simulink model "edma_scatter_gather_transfer_s32k14x"  (Simulink 9.0)
settings: Solver=FixedStepDiscrete  StartTime=0.0  StopTime=10.0  FixedStep=0.5  RelTol=1e-3  EnableMultiTasking=on
InitFcn:
  | mbd_s32k_consistency_checks(bdroot(gcs));
undefined symbols (not defined in the file): LQFP
libraries: mbd_s32k1xx_ec_toolbox x6, simulink x1
Description:
  | Press SW3 to trigger an eDMA transfer to PTOR register; this toggles PTD0 and PTD15,
  | thus blinking the red and blue LEDs.
  | 
  | Press SW2 to trigger eDMA transfer continuously (at every step). Pressing it again will stop this process.
  | 
  | Verification:
  | LED blink (purple) at every SW3 press.
  | LED blinks continuously at 0.5s after pressing SW2.
settings Model: Creator=NXP MBDT Team  LastModifiedBy=nxf35172
settings DataIOCC: ExternalInput=off  InitialState=off  LimitDataPoints=on  SaveFormat=Dataset  SaveOutput=off  SignalLogging=off  SaveTime=off
settings OptimizationCC: DefaultParameterBehavior=Inlined  PassReuseOutputArgsAs=Individual arguments  LifeSpan=auto
settings DebuggingCC: UnderspecifiedInitializationDetection=Simplified  MergeDetectMultiDrivingBlocksExec=error  InheritedTsInSrcMsg=none  SingleTaskRateTransMsg=error  ParameterTunabilityLossMsg=error  UnconnectedInputMsg=error  UnconnectedOutputMsg=error  UnconnectedLineMsg=error  AllowSymbolicDim=off  UnknownTsInhSupMsg=error
settings HardwareCC: ProdLargestAtomicInteger=Long  ProdLargestAtomicFloat=Double  ProdIntDivRoundTo=Zero  ProdEndianess=LittleEndian  ProdHWDeviceType=ARM Compatible->ARM Cortex
settings SFSimCC: MATLABDynamicMemAlloc=off
settings RTWCC: SystemTargetFile=mbd_s32k.tlc  MakeCommand=mbd_s32k_make_rtw COPY_MDLREF_INCLUDES=0  TemplateMakefile=mbd_s32k.tmf  Description=Model Based Design Toolbox S32K14x Code Generation Target  GenerateReport=on  IncludeHyperlinkInReport=on  LaunchReport=on  GenerateTraceInfo=on  GenerateTraceReport=on  GenerateTraceReportSl=on  GenerateTraceReportSf=on  GenerateTraceReportEml=on
settings CodeAppCC: ForceParamTrailComments=on  IgnoreCustomStorageClasses=off  OperatorAnnotations=on  SimulinkDataObjDesc=on  SFDataObjDesc=on  InsertBlockDesc=on  StateflowObjectComments=off
settings STFCustomTargetCC: MultiwordLength=256  ModelReferenceCompliant=off  CombineOutputUpdateFcns=on  ERTCustomFileBanners=on  SupportContinuousTime=off  SupportNonInlinedSFcns=off  RemoveResetFunc=on  MATLABClassNameForMDSCustomization=Simulink.SoftwareTarget.ERTCustomization  GRTInterface=off  SystemTargetFile=mbd_s32k.tlc
settings ERTTargetCC: ModelReferenceCompliant=off  ParMdlRefBuildCompliant=off  CompOptLevelCompliant=off  ConcurrentExecutionCompliant=off  ModelStepFunctionPrototypeControlCompliant=off  CPPClassGenCompliant=off  UseToolchainInfoCompliant=off  InlinedParameterPlacement=NonHierarchical  ERTCustomFileTemplate=example_file_process.tlc

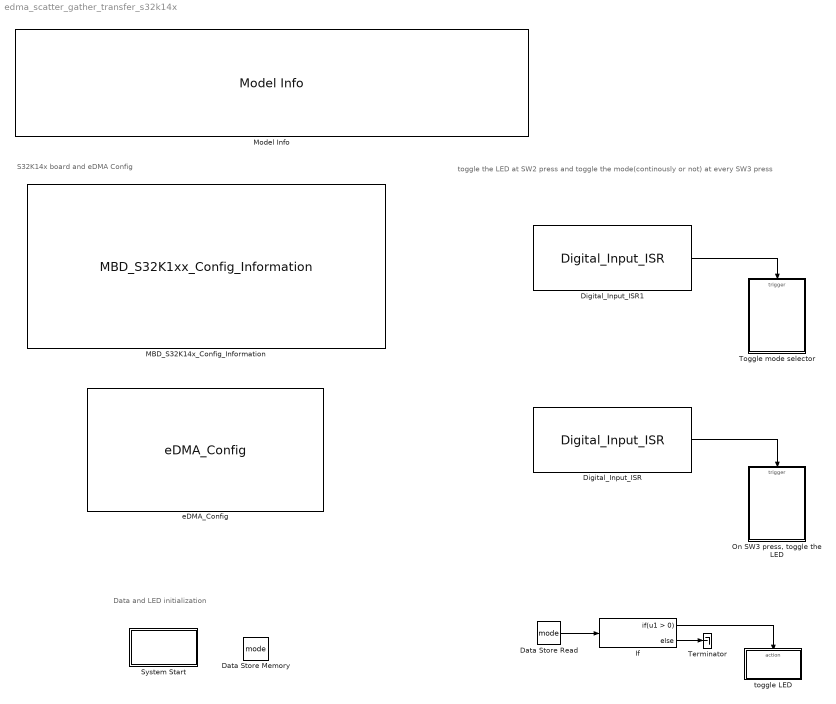
== system edma_scatter_gather_transfer_s32k14x ==
  note: toggle the LED at SW2 press and toggle the mode(continously or not) at every SW3 press
  note: S32K14x board and eDMA Config
  note: Data and LED initialization
  Data Store Memory : DataStoreMemory  DataStoreName=mode  ReadBeforeWriteMsg=warning  WriteAfterWriteMsg=warning  WriteAfterReadMsg=warning  ShowAdditionalParam=off
  Data Store Read : DataStoreRead  DataStoreName=mode
  Digital_Input_ISR : mbd_s32k1xx_ec_toolbox/GPIO Blocks/Digital_Input_ISR  gpio_pin=PTC13: [PTC13 | Port C I/O]  irqc=on rising-edge  prio=15
  Digital_Input_ISR1 : mbd_s32k1xx_ec_toolbox/GPIO Blocks/Digital_Input_ISR  gpio_pin=PTC12: [PTC12 | Port C I/O]  irqc=on rising-edge  prio=15
  If : If
  MBD_S32K14x_Config_Information : mbd_s32k1xx_ec_toolbox/MBD_S32K1xx_Config_Information  mbdt_ver=0  disp_str=|  config_params=[]  mcu_target_name=S32K144  mcu_target_package=100-LQFP  mcu_target_sram_size=64KB  mcu_system_clock_freq=80  mcu_xtal_freq=External 8  mcu_steptick_timer=LPIT Channel 0  mcu_steptick_prio=15  ds_import_enable=on  target_compiler=GCC  target_memory=FLASH  gcc_target_compile_opts=-mcpu=cortex-m4 -mthumb -mfloat-abi=hard -mfpu=fpv4-sp-d16 -O1 -g -gstrict-dwarf  gcc_target_assemble_opts=-mcpu=cortex-m4 -mthumb -mfloat-abi=hard -mfpu=fpv4-sp-d16 -g  gcc_target_link_opts=-mcpu=cortex-m4 -mthumb -mfloat-abi=hard -mfpu=fpv4-sp-d16  gcc_target_default_lcf=on  gcc_target_user_lcf=S32K144_64_flash.ld  ghs_target_compile_opts=-cpu=cortexm4f -thumb -DARM_MATH_CM4 -fpu=vfpv4_d16 -fsingle -Ogeneral -Wundef -Wimplicit-int -Wshadow -Wtrigraphs --no_commons --gnu_asm -gnu99 -gdwarf-2 -G  ghs_target_assemble_opts=-cpu=cortexm4f -fpu=vfpv4_d16  ghs_target_link_opts=-cpu=cortexm4f -thumb -fpu=vfpv4_d16  ghs_target_default_lcf=off  ghs_target_user_lcf=S32K144_64_flash.ld  iar_target_compile_opts=--cpu=Cortex-M4F --thumb --fpu=VFPv4_sp -Ol -e --debug --dlib_config normal  iar_target_assemble_opts=--cpu Cortex-M4F --thumb --fpu VFPv4_sp  iar_target_link_opts=--no_exceptions --vfe --inline  iar_target_default_lcf=off  iar_target_user_lcf=S32K144_64_flash.icf  pil_download_enable=off  rbl_download_enable=on  rbl_start_delay=5000000  rbl_download_interface=OpenSDA  rbl_restart_request=off  rbl_com_port=Custom  rbl_com_port_custom=COM1  pil_download_rate=57600  pil_opensda_drive=Custom  pil_opensda_drive_custom=D  pil_uart_instance=0  pil_uart_rx=PTA2: [LPUART0_RX | Receive]  pil_uart_tx=PTA3: [LPUART0_TX | Transmit]  FTM_PWM_PcrCheckEnDis=on  FTM_Input_Edge_Inputs_PcrCheckEnDis=on  FTM_Dual_Edge_Inputs_PcrCheckEnDis=on  FTM_Quadrature_Inputs_PcrCheckEnDis=on  FTM_Hall_Sensor_Inputs_PcrCheckEnDis=on  LPTMR_PcrCheckEnDis=on  PIT_PcrCheckEnDis=on  RTC_PcrCheckEnDis=on  FlexCAN_PcrCheckEnDis=on  LIN_PcrCheckEnDis=on  FlexIO_PcrCheckEnDis=on  LPI2C_PcrCheckEnDis=on  LPSPI_PcrCheckEnDis=on  LPUART_PcrCheckEnDis=on  CMP_PcrCheckEnDis=on  GPIO_OutputPcrCheckEnDis=on  GPIO_InputPcrCheckEnDis=on  SBC_PcrCheckEnDis=on  AMMCLIB_PcrCheckEnDis=on  FM_PcrCheckEnDis=on  Profile_PcrCheckEnDis=on  ConfigParams_PcrCheckEnDis=on  ModelRef_PcrCheckEnDis=on  PDB0_PcrCheckEnDis=on  CSEc_PcrCheckEnDis=on  eDMA_PcrCheckEnDis=on  ADC_PcrCheckEnDis=on  WDOG_PcrCheckEnDis=on
      | Target : S32K144-64KB_SRAM
      | Package : 100-pin
      | System clock : 80 MHz
      | XTAL clock : External 8 MHz
      | Compiler : GreenHills Multi
      | Target Type : FLASH
      | Download Code after build : (OpenSDA: F)
      | Step Tick Interrupt Priority : 15
  Model Info : simulink/Model-Wide Utilities/Model Info  Frame=off  DisplayStringWithTags=|  HorizontalTextAlignment=Left  LeftAlignmentValue=0.02
      | Model Name: %<ModelName>
      | 
      | Description: %<Description>
  "On SW3 press, toggle the LED" : Subsystem
  System Start : Subsystem  mask(System Start){ShowInLibBrowser=0}
      mask prompts: ShowInLibBrowser "Simulink:masks:CustCodeMaskParam1_MP"
      settings: CopyFcn=cccopyfcn(gcb)  OpenFcn=ccopenfcn('System Start Function')
      mask Help: eval('feval(''rtwprivate'',''rtwhelpview'',''rtw_sys_start_block'')');
      mask Display: disp('Initialize\nLEDs');
  Terminator : Terminator
  Toggle mode selector : Subsystem
  eDMA_Config : mbd_s32k1xx_ec_toolbox/Core and System Blocks/DMA Blocks/eDMA_Config  channel=0  show_advanced_tab=on  channel_advanced_checkbox=on  show_enabled=on  arbitration=EDMA_ARBITRATION_FIXED_PRIORITY  halt_on_error=false  channel0priority=EDMA_CHN_DEFAULT_PRIORITY  channel0requestsource=EDMA_REQ_DISABLED  channel0enable=on  channel1priority=EDMA_CHN_DEFAULT_PRIORITY  channel1requestsource=EDMA_REQ_DISABLED  channel1enable=off  channel2priority=EDMA_CHN_DEFAULT_PRIORITY  channel2requestsource=EDMA_REQ_DISABLED  channel2enable=off  channel3priority=EDMA_CHN_DEFAULT_PRIORITY  channel3requestsource=EDMA_REQ_DISABLED  channel3enable=off  channel4priority=EDMA_CHN_DEFAULT_PRIORITY  channel4requestsource=EDMA_REQ_DISABLED  channel4enable=off  channel5priority=EDMA_CHN_DEFAULT_PRIORITY  channel5requestsource=EDMA_REQ_DISABLED  channel5enable=off  channel6priority=EDMA_CHN_DEFAULT_PRIORITY  channel6requestsource=EDMA_REQ_DISABLED  channel6enable=off  channel7priority=EDMA_CHN_DEFAULT_PRIORITY  channel7requestsource=EDMA_REQ_DISABLED  channel7enable=off  channel8priority=EDMA_CHN_DEFAULT_PRIORITY  channel8requestsource=EDMA_REQ_DISABLED  channel8enable=off  channel9priority=EDMA_CHN_DEFAULT_PRIORITY  channel9requestsource=EDMA_REQ_DISABLED  channel9enable=off  channel10priority=EDMA_CHN_DEFAULT_PRIORITY  channel10requestsource=EDMA_REQ_DISABLED  channel10enable=off  channel11priority=EDMA_CHN_DEFAULT_PRIORITY  channel11requestsource=EDMA_REQ_DISABLED  channel11enable=off  channel12priority=EDMA_CHN_DEFAULT_PRIORITY  channel12requestsource=EDMA_REQ_DISABLED  channel12enable=off  channel13priority=EDMA_CHN_DEFAULT_PRIORITY  channel13requestsource=EDMA_REQ_DISABLED  channel13enable=off  channel14priority=EDMA_CHN_DEFAULT_PRIORITY  channel14requestsource=EDMA_REQ_DISABLED  channel14enable=off  channel15priority=EDMA_CHN_DEFAULT_PRIORITY  channel15requestsource=EDMA_REQ_DISABLED  channel15enable=off
  toggle LED : Subsystem  TreatAsAtomicUnit=on
  wires:
  Digital_Input_ISR/1 -> "On SW3 press, toggle the LED"/Trigger
  Digital_Input_ISR1/1 -> Toggle mode selector/Trigger
  If/1 -> toggle LED/Action
  Data Store Read/1 -> If/1
  If/2 -> Terminator/1

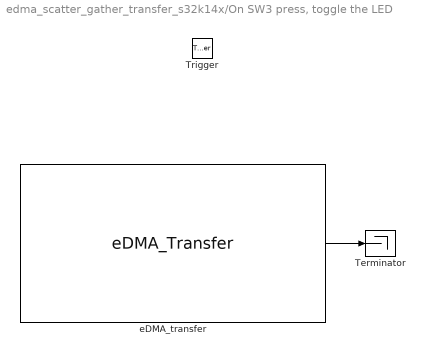
== system edma_scatter_gather_transfer_s32k14x/On SW3 press, toggle the LED ==
  Trigger : TriggerPort  TriggerType=function-call  VariantControl=Variant  PortDimensions=1
  Terminator : Terminator
  eDMA_transfer : mbd_s32k1xx_ec_toolbox/Core and System Blocks/DMA Blocks/eDMA_Transfer  channel=0  transfer_mode=Scatter-Gather Transfer  transfer_type=EDMA_TRANSFER_MEM2PERIPH  transfer_size=EDMA_TRANSFER_SIZE_4B  single_block_src_type=Src input is an address  single_block_dest_type=Dest input is an address  bytes_on_each_req=4  sg_struct_size=32  src_list={32769}  src_list_type=Value list  dest_list={0x0,0x0}  dest_list_type=Select from a register list  src_periph1=ADC0  src_reg1=SC1C  src_reg1offset=0xABh  src_reg1enable=on  src_reg1_addr=0x4003B008  src_periph2=ADC0  src_reg2=SC1A  src_reg2offset=0  src_reg2enable=on  src_reg2_addr=0x4003B000  src_periph3=ADC0  src_reg3=SC1A  src_reg3offset=17  src_reg3enable=on  src_reg3_addr=0x4003B000  src_periph4=ADC0  src_reg4=SC1A  src_reg4offset=0  src_reg4enable=off  src_reg4_addr=0x4003B000  src_periph5=ADC0  src_reg5=SC1A  src_reg5offset=0  src_reg5enable=off  src_reg5_addr=0x4003B000  src_periph6=ADC0  src_reg6=SC1A  src_reg6offset=0  src_reg6enable=off  src_reg6_addr=0x4003B000  src_periph7=ADC0  src_reg7=SC1A  src_reg7offset=0  src_reg7enable=off  src_reg7_addr=0x4003B000  src_periph8=ADC0  src_reg8=SC1A  src_reg8offset=0  src_reg8enable=off  src_reg8_addr=0x4003B000  dest_periph1=PTD  dest_reg1=PDOR  dest_reg1offset=0xCh  dest_reg1enable=on  dest_reg1_addr=0x400FF0C0  dest_periph2=ADC0  dest_reg2=SC1A  dest_reg2offset=abch  dest_reg2enable=off  dest_reg2_addr=0x4003B000  dest_periph3=ADC0  dest_reg3=SC1A  dest_reg3offset=0xabcd  dest_reg3enable=off  dest_reg3_addr=0x4003B000  dest_periph4=ADC0  dest_reg4=SC1A  dest_reg4offset=0  dest_reg4enable=off  dest_reg4_addr=0x4003B000  dest_periph5=ADC0  dest_reg5=SC1A  dest_reg5offset=0  dest_reg5enable=off  dest_reg5_addr=0x4003B000  dest_periph6=ADC0  dest_reg6=SC1A  dest_reg6offset=0  dest_reg6enable=off  dest_reg6_addr=0x4003B000  dest_periph7=ADC0  dest_reg7=SC1A  dest_reg7offset=0  dest_reg7enable=off  dest_reg7_addr=0x4003B000  dest_periph8=ADC0  dest_reg8=SC1A  dest_reg8offset=0  dest_reg8enable=off  dest_reg8_addr=0x4003B000
  wires:
  eDMA_transfer/1 -> Terminator/1

== system edma_scatter_gather_transfer_s32k14x/System Start ==

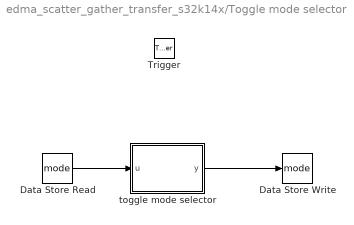
== system edma_scatter_gather_transfer_s32k14x/Toggle mode selector ==
  Trigger : TriggerPort  TriggerType=function-call  VariantControl=Variant  PortDimensions=1
  Data Store Read : DataStoreRead  DataStoreName=mode
  Data Store Write : DataStoreWrite  DataStoreName=mode
  toggle mode selector : MATLAB Function  TreatAsAtomicUnit=on
  wires:
  toggle mode selector/1(y) -> Data Store Write/1
  Data Store Read/1 -> toggle mode selector/1(u)

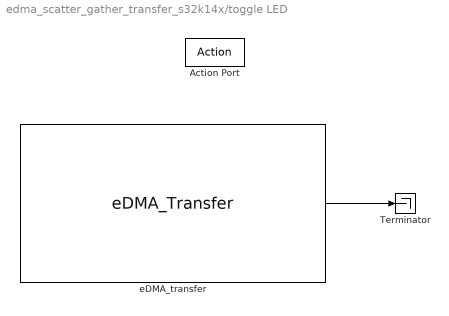
== system edma_scatter_gather_transfer_s32k14x/toggle LED ==
  Action Port : ActionPort
  Terminator : Terminator
  eDMA_transfer : mbd_s32k1xx_ec_toolbox/Core and System Blocks/DMA Blocks/eDMA_Transfer  channel=0  transfer_mode=Scatter-Gather Transfer  transfer_type=EDMA_TRANSFER_MEM2PERIPH  transfer_size=EDMA_TRANSFER_SIZE_4B  single_block_src_type=Src input is an address  single_block_dest_type=Dest input is an address  bytes_on_each_req=4  sg_struct_size=32  src_list={32769}  src_list_type=Value list  dest_list={PTD_BASE + 0xc, 0x400FF0CC}  dest_list_type=Select from a register list  src_periph1=ADC0  src_reg1=SC1C  src_reg1offset=0xABh  src_reg1enable=on  src_reg1_addr=0x4003B008  src_periph2=ADC0  src_reg2=SC1A  src_reg2offset=0  src_reg2enable=on  src_reg2_addr=0x4003B000  src_periph3=ADC0  src_reg3=SC1A  src_reg3offset=17  src_reg3enable=on  src_reg3_addr=0x4003B000  src_periph4=ADC0  src_reg4=SC1A  src_reg4offset=0  src_reg4enable=off  src_reg4_addr=0x4003B000  src_periph5=ADC0  src_reg5=SC1A  src_reg5offset=0  src_reg5enable=off  src_reg5_addr=0x4003B000  src_periph6=ADC0  src_reg6=SC1A  src_reg6offset=0  src_reg6enable=off  src_reg6_addr=0x4003B000  src_periph7=ADC0  src_reg7=SC1A  src_reg7offset=0  src_reg7enable=off  src_reg7_addr=0x4003B000  src_periph8=ADC0  src_reg8=SC1A  src_reg8offset=0  src_reg8enable=off  src_reg8_addr=0x4003B000  dest_periph1=PTD  dest_reg1=PDOR  dest_reg1offset=0xCh  dest_reg1enable=on  dest_reg1_addr=0x400FF0C0  dest_periph2=ADC0  dest_reg2=SC1A  dest_reg2offset=abch  dest_reg2enable=off  dest_reg2_addr=0x4003B000  dest_periph3=ADC0  dest_reg3=SC1A  dest_reg3offset=0xabcd  dest_reg3enable=off  dest_reg3_addr=0x4003B000  dest_periph4=ADC0  dest_reg4=SC1A  dest_reg4offset=0  dest_reg4enable=off  dest_reg4_addr=0x4003B000  dest_periph5=ADC0  dest_reg5=SC1A  dest_reg5offset=0  dest_reg5enable=off  dest_reg5_addr=0x4003B000  dest_periph6=ADC0  dest_reg6=SC1A  dest_reg6offset=0  dest_reg6enable=off  dest_reg6_addr=0x4003B000  dest_periph7=ADC0  dest_reg7=SC1A  dest_reg7offset=0  dest_reg7enable=off  dest_reg7_addr=0x4003B000  dest_periph8=ADC0  dest_reg8=SC1A  dest_reg8offset=0  dest_reg8enable=off  dest_reg8_addr=0x4003B000
  wires:
  eDMA_transfer/1 -> Terminator/1

== matlab function Toggle mode selector/toggle mode selector ==
  data: u input double; y output double
function y = fcn(u)
%#codegen

if u==0
    y=1;
else
    y=0;
end
